simulink model "TCS5"  (R2018b)
settings: Solver=VariableStepAuto  StartTime=0.0  StopTime=10  RelTol=1e-3
model workspace (MAT data in the model file):
  Ki = Simulink.Parameter
  Ki.Value = 50000
  Ki.Description = 'PID积分系数'
  Ki.DataType = 'auto'
  Ki.Dimensions = [1 1]
  Kp = Simulink.Parameter
  Kp.Value = 40000
  Kp.Description = 'PID比例系数'
  Kp.DataType = 'auto'
  Kp.Dimensions = [1 1]
  T_max = Simulink.Parameter
  T_max.Value = 10000
  T_max.Description = '电机最大转矩'
  T_max.DataType = 'auto'
  T_max.Dimensions = [1 1]
  Vobj = Simulink.Parameter
  Vobj.Value = 40
  Vobj.DataType = 'auto'
  Vobj.Dimensions = [1 1]
  r = Simulink.Parameter
  r.Value = 0.538
  r.Description = '车轮滚动半径'
  r.DataType = 'auto'
  r.Dimensions = [1 1]
  s_obj = Simulink.Parameter
  s_obj.Value = 0.13
  s_obj.DataType = 'auto'
  s_obj.Dimensions = [1 1]
undefined symbols (not defined in the file): DiscIntNeverNeededParam
libraries: simulink x8, Solver_SF x1
(part 1 of 2)
settings Model: OrderedModelArguments=off  Creator=14615  LastModifiedBy=14615
settings DataIOCC: ReturnWorkspaceOutputs=on
settings DebuggingCC: SFMachineParentedDataDiag=error

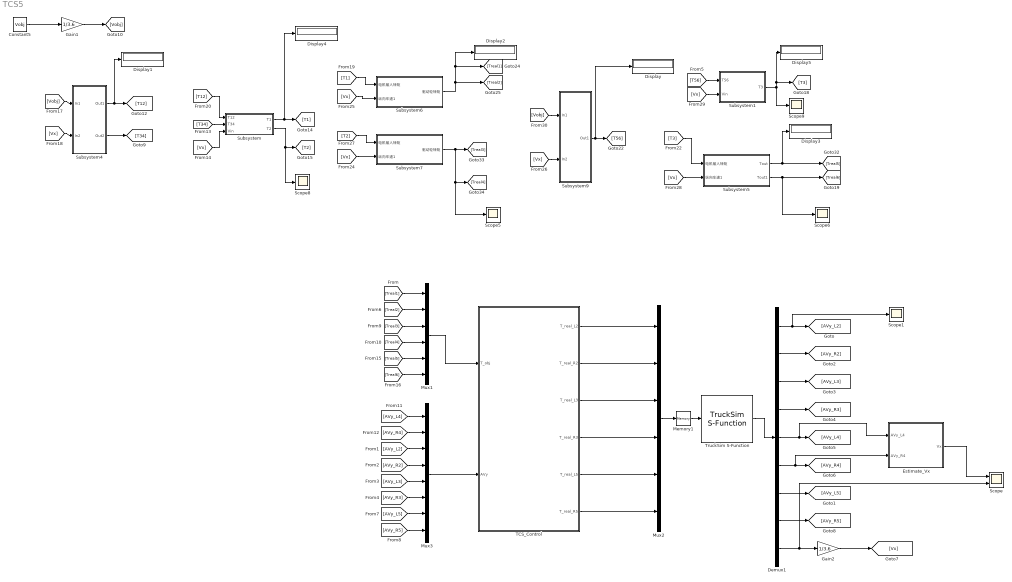
== system TCS5 ==
  Constant5 : Constant  Value=Vobj
  Demux1 : Demux  Outputs=9
  Display{,1..5} (6 alike) : Display
  Estimate_Vx : Subsystem
  Gain1 : Gain  Gain=1/3.6
  Gain2 : Gain  Gain=1/3.6
  Memory1 : Memory
  Mux1 : Mux  Inputs=6
  Mux2 : Mux  Inputs=6
  Mux3 : Mux  Inputs=8
  Scope : Scope  NumInputPorts=2
  Scope{1,5..6,8..9} (5 alike) : Scope
  Subsystem : Subsystem
  Subsystem1 : Subsystem
  Subsystem4 : Subsystem
  Subsystem5 : Subsystem
  Subsystem6 : Subsystem
  Subsystem7 : Subsystem
  Subsystem9 : Subsystem
  TCS_Control : Subsystem
  TruckSim S-Function : Solver_SF/TruckSim S-Function  Priority=1  SIMFILE=simfile.sim
  wires:
  Mux1/1 -> TCS_Control/1(T_obj)
  Mux2/1 -> Memory1/1
  TruckSim S-Function/1 -> Demux1/1
  Memory1/1 -> TruckSim S-Function/1
  Mux3/1 -> TCS_Control/2(AVy)
  [Treal1] -> Mux1/1
  [Treal6] -> Mux1/6
  [Treal4] -> Mux1/4
  [Treal3] -> Mux1/3
  [Treal2] -> Mux1/2
  [Treal5] -> Mux1/5
  [AVy_L4] -> Mux3/1
  [AVy_R4] -> Mux3/2
  [AVy_L2] -> Mux3/3
  [AVy_R2] -> Mux3/4
  [AVy_L3] -> Mux3/5
  [AVy_R3] -> Mux3/6
  [AVy_L5] -> Mux3/7
  [AVy_R5] -> Mux3/8
  TCS_Control/2(T_real_R2) -> Mux2/2
  TCS_Control/3(T_real_L3) -> Mux2/3
  TCS_Control/1(T_real_L2) -> Mux2/1
  TCS_Control/4(T_real_R3) -> Mux2/4
  Demux1/8 -> [AVy_R5]
  Demux1/6 -> Estimate_Vx/2(AVy_R4), [AVy_R4]
  Demux1/9 -> Scope/2, Gain2/1
  Estimate_Vx/1(Vx) -> Scope/1
  TCS_Control/5(T_real_L5) -> Mux2/5
  TCS_Control/6(T_real_R5) -> Mux2/6
  Subsystem/1(T1) -> Display4/1, [T1]
  [T1] -> Subsystem6/1(电机输入转矩)
  [Vobj] -> Subsystem9/1(In1)
  [T12] -> Subsystem/1(T12)
  Subsystem6/1(驱动轮转矩) -> [Treal2], [Treal1], Display2/1
  [T2] -> Subsystem7/1(电机输入转矩)
  [T3] -> Subsystem5/1(电机输入转矩)
  [Vobj] -> Subsystem4/1(In1)
  [T34] -> Subsystem/2(T34)
  Subsystem5/1(Tout) -> Display3/1, [Treal5]
  Subsystem4/1(Out1) -> Display1/1, [T12]
  Subsystem9/1(Out1) -> Display/1, [T56]
  [Vx] -> Subsystem4/2(In2)
  [T56] -> Subsystem1/1(T56)
  Subsystem/2(T2) -> Scope8/1, [T2]
  Subsystem4/2(Out2) -> [T34]
  Subsystem5/2(Tout1) -> [Treal6], Scope6/1
  Subsystem7/1(驱动轮转矩) -> [Treal4], Scope5/1, [Treal3]
  [Vx] -> Subsystem7/2(纵向车速1)
  [Vx] -> Subsystem1/2(Vin)
  [Vx] -> Subsystem9/2(In2)
  [Vx] -> Subsystem/3(Vin)
  Constant5/1 -> Gain1/1
  Subsystem1/1(T3) -> Display5/1, [T3], Scope9/1
  [Vx] -> Subsystem6/2(纵向车速1)
  [Vx] -> Subsystem5/2(纵向车速1)
  Gain1/1 -> [Vobj]
  Gain2/1 -> [Vx]
  Demux1/1 -> Scope1/1, [AVy_L2]
  Demux1/2 -> [AVy_R2]
  Demux1/3 -> [AVy_L3]
  Demux1/4 -> [AVy_R3]
  Demux1/5 -> Estimate_Vx/1(AVy_L4), [AVy_L4]
  Demux1/7 -> [AVy_L5]

== system TCS5/Estimate_Vx ==
  AVy_L4 : Inport
  AVy_R4 : Inport  Port=2
  Add : Sum
  Gain : Gain  Gain=pi/30
  Gain1 : Gain  Gain=3.6
  Gain2 : Gain  Gain=pi/30
  Gain3 : Gain  Gain=3.6
  Gain4 : Gain  Gain=0.5
  Product : Product
  Product1 : Product
  轮胎滚动半径 : Constant  Value=r
  轮胎滚动半径1 : Constant  Value=r
  Vx : Outport
  wires:
  Gain/1 -> Product/1
  Product1/1 -> Gain3/1
  Gain3/1 -> Add/2
  轮胎滚动半径/1 -> Product/2
  轮胎滚动半径1/1 -> Product1/2
  Add/1 -> Gain4/1
  Gain4/1 -> Vx/1
  Product/1 -> Gain1/1
  Gain1/1 -> Add/1
  Gain2/1 -> Product1/1
  AVy_R4/1 -> Gain2/1
  AVy_L4/1 -> Gain/1

== system TCS5/Subsystem ==
  T12 : Inport
  T34 : Inport  Port=2
  Vin : Inport  Port=3
  Gain : Gain  Gain=3.6
  Product : Product  SaturateOnIntegerOverflow=on  InputSameDT=on  OutDataTypeStr=Inherit: Same as first input
  Product1 : Product  SaturateOnIntegerOverflow=on  InputSameDT=on  OutDataTypeStr=Inherit: Same as first input
  Saturation : Saturate  UpperLimit=2000  LowerLimit=-2000
  Saturation1 : Saturate  UpperLimit=2000  LowerLimit=-2000
  Table : Lookup_n-D  NumberOfTableDimensions=1  BreakpointsForDimension1=[1 2 3 4]  Table=[0.1261,0.2833,0.5747,1.00]  OutDataTypeStr=double  SaturateOnIntegerOverflow=on  InputSameDT=on  LockScale=on
  换挡逻辑 : Subsystem
  T1 : Outport  VectorParamsAs1DForOutWhenUnconnected=on
  T2 : Outport  Port=2  VectorParamsAs1DForOutWhenUnconnected=on
  wires:
  Vin/1 -> Gain/1
  换挡逻辑/1(gear) -> Table/1
  T12/1 -> Product/1
  Table/1 -> Product/2, Product1/1
  T34/1 -> Product1/2
  Gain/1 -> 换挡逻辑/1(v)
  Product1/1 -> Saturation/1
  Saturation/1 -> T2/1
  Product/1 -> Saturation1/1
  Saturation1/1 -> T1/1

== system TCS5/Subsystem1 ==
  T56 : Inport
  Vin : Inport  Port=2
  Gain : Gain  Gain=3.6
  Gain2 : Gain
  Product2 : Product  SaturateOnIntegerOverflow=on  InputSameDT=on  OutDataTypeStr=Inherit: Same as first input
  Saturation1 : Saturate  UpperLimit=2000  LowerLimit=-2000
  Table : Lookup_n-D  NumberOfTableDimensions=1  BreakpointsForDimension1=[1 2 3 4]  Table=[0.1261,0.2833,0.5747,1.00]  OutDataTypeStr=double  SaturateOnIntegerOverflow=on  InputSameDT=on  LockScale=on
  换挡逻辑 : Subsystem
  T3 : Outport  VectorParamsAs1DForOutWhenUnconnected=on
  wires:
  换挡逻辑/1(gear) -> Table/1
  Vin/1 -> Gain/1
  Table/1 -> Product2/1
  T56/1 -> Product2/2
  Gain/1 -> 换挡逻辑/1(v)
  Product2/1 -> Saturation1/1
  Saturation1/1 -> Gain2/1
  Gain2/1 -> T3/1

== system TCS5/Subsystem4 ==
  In1 : Inport
  In2 : Inport  Port=2
  0.1 : simulink/Continuous/PID Controller  Controller=PID  Form=Parallel  TimeDomain=Discrete-time  SampleTime=-1  IntegratorMethod=Forward Euler  FilterMethod=Forward Euler  ControllerParametersSource=internal  P=10000  I=0  D=0  UseFilter=on  N=100  TunerSelectOption=Transfer Function Based (PID Tuner App)  InitialConditionSource=internal  InitialConditionForIntegrator=0  InitialConditionForFilter=0  DifferentiatorICPrevScaledInput=0  ExternalReset=none  TrackingMode=off  Kt=1  LimitOutput=off  UpperSaturationLimit=inf  LowerSaturationLimit=-inf  LinearizeAsGain=on  AntiWindupMode=none  Kb=1  POutMin=[]  POutMax=[]  IOutMin=[]  IOutMax=[]  DOutMin=[]  DOutMax=[]  NOutMin=[]  NOutMax=[]  SumOutMin=[]  SumOutMax=[]  SaturationOutMin=[]  SaturationOutMax=[]  PParamMin=[]  PParamMax=[]  IParamMin=[]  IParamMax=[]  DParamMin=[]  DParamMax=[]  NParamMin=[]  NParamMax=[]  KbParamMin=[]  KbParamMax=[]  KtParamMin=[]  KtParamMax=[]  KbOutMin=[]  KbOutMax=[]  KtOutMin=[]  KtOutMax=[]  IntegratorOutMin=[]  IntegratorOutMax=[]  FilterOutMin=[]  FilterOutMax=[]  SumI1OutMin=[]  SumI1OutMax=[]  SumI2OutMin=[]  SumI2OutMax=[]  SumI3OutMin=[]  SumI3OutMax=[]  SumI4OutMin=[]  SumI4OutMax=[]  SumDOutMin=[]  SumDOutMax=[]  DifferentiatorOutMin=[]  DifferentiatorOutMax=[]  FilterDiffOutCoefMin=[]  FilterDiffOutCoefMax=[]  ReciprocalOutMin=[]  ReciprocalOutMax=[]  SumDenOutMin=[]  SumDenOutMax=[]  SumNumOutMin=[]  SumNumOutMax=[]  DivideOutMin=[]  DivideOutMax=[]  IntegratorContinuousStateAttributes=''  IntegratorStateMustResolveToSignalObject=off  IntegratorRTWStateStorageClass=Auto  FilterContinuousStateAttributes=''  FilterStateMustResolveToSignalObject=off  FilterRTWStateStorageClass=Auto  ParallelPVariant=InternalParameters  IdealPVariant=Disabled  IVariant=InternalParameters  DVariant=InternalParameters  IntegratorVariant=Discrete  SatVariant=Disabled  AWVariant=Passthrough  PCopyVariant=Disabled  TRVariant=Disabled  FdbkBlocksVariant=Forward  IdealPFdbkVariant=Disabled  SatFdbkVariant=Disabled  DerivativeFilterVariant=ForwardEulerFilter  NVariant=InternalParameters  NCopyVariant=Disabled  FilterICVariant=InternalICsFilter  IntegratorICVariant=InternalICs  ExternalResetVariant=Disabled  TRSumVariant=Passthrough  SumFdbkVariant=Disabled  SumVariant=Sum_PID
  Fcn : Fcn  Expr=u(1)*u(2)/4
  Mux : Mux  Inputs=2
  R : Constant  Value=0.538
  Sum : Sum  Inputs=|+-
  Out1 : Outport  VectorParamsAs1DForOutWhenUnconnected=on
  Out2 : Outport  Port=2  VectorParamsAs1DForOutWhenUnconnected=on
  wires:
  0.1/1 -> Mux/1
  Fcn/1 -> Out2/1, Out1/1
  Sum/1 -> 0.1/1
  In1/1 -> Sum/1
  In2/1 -> Sum/2
  R/1 -> Mux/2
  Mux/1 -> Fcn/1

== system TCS5/Subsystem5 ==
  电机输入转矩 : Inport
  纵向车速1 : Inport  Port=2
  Gain : Gain  Gain=3.6
  PMSM : Subsystem  mask{pp=4, Rs=0.05, Jm=0.008, ld=0.0001, lq=0.0001, flux=0.17, f=1.349e-5}
      mask prompts: pp "极对数"; Rs "定子电阻"; Jm "转动惯量"; ld "d轴电感"; lq "q轴电感"; flux "永磁体磁链"; f "粘性阻尼"
  Product : Product
  SOC : Scope
  Subsystem : Subsystem
  充电电流 : Scope
  单位三相电 : Sin  Frequency=400*pi  Phase=[0 -2*pi/3 2*pi/3]  SampleTime=0
  变速器模型 : Subsystem
  差速器 : Gain  Gain=1/2
  换挡逻辑 : Subsystem
  电机输入\输出转矩 : Scope  NumInputPorts=2
  能量变化 : Scope
  驱动轮的转矩 : Scope
  Tout : Outport  VectorParamsAs1DForOutWhenUnconnected=on
  Tout1 : Outport  Port=2  VectorParamsAs1DForOutWhenUnconnected=on
  wires:
  差速器/1 -> Tout1/1, Tout/1, 驱动轮的转矩/1
  电机输入转矩/1 -> 电机输入\输出转矩/1, PMSM/1(Tm)
  换挡逻辑/1(gear) -> 变速器模型/2(Gear)
  变速器模型/1(Tout) -> 差速器/1
  Subsystem/1(能量变化) -> 能量变化/1
  PMSM/1(Te) -> 电机输入\输出转矩/2, 变速器模型/1(Tin)
  纵向车速1/1 -> Gain/1
  Product/1 -> PMSM/2(Uabc)
  单位三相电/1 -> Product/2
  Subsystem/3(输出电压V) -> Product/1
  PMSM/2(iq) -> 充电电流/1, Subsystem/1(充电电流A)
  Subsystem/2(SOC) -> SOC/1
  Gain/1 -> 换挡逻辑/1(v)

== system TCS5/Subsystem6 ==
  电机输入转矩 : Inport
  纵向车速1 : Inport  Port=2
  Gain : Gain  Gain=3.6
  PMSM : Subsystem  mask{pp=4, Rs=0.05, Jm=0.008, ld=0.0001, lq=0.0001, flux=0.17, f=1.349e-5}
      mask prompts: pp "极对数"; Rs "定子电阻"; Jm "转动惯量"; ld "d轴电感"; lq "q轴电感"; flux "永磁体磁链"; f "粘性阻尼"
  Product : Product
  SOC : Scope
  Subsystem : Subsystem
  充电电流 : Scope
  单位三相电 : Sin  Frequency=400*pi  Phase=[0 -2*pi/3 2*pi/3]  SampleTime=0
  变速器模型 : Subsystem
  差速器 : Gain  Gain=1/2
  换挡逻辑 : Subsystem
  能量变化 : Scope
  驱动轮的转矩 : Scope
  驱动轮转矩 : Outport  VectorParamsAs1DForOutWhenUnconnected=on
  wires:
  Product/1 -> PMSM/2(Uabc)
  电机输入转矩/1 -> PMSM/1(Tm)
  变速器模型/1(Tout) -> 差速器/1
  Subsystem/2(SOC) -> SOC/1
  纵向车速1/1 -> Gain/1
  换挡逻辑/1(gear) -> 变速器模型/2(Gear)
  PMSM/1(Te) -> 变速器模型/1(Tin)
  Subsystem/3(输出电压V) -> Product/1
  单位三相电/1 -> Product/2
  PMSM/2(iq) -> 充电电流/1, Subsystem/1(充电电流A)
  差速器/1 -> 驱动轮的转矩/1, 驱动轮转矩/1
  Subsystem/1(能量变化) -> 能量变化/1
  Gain/1 -> 换挡逻辑/1(v)

== system TCS5/Subsystem7 ==
  电机输入转矩 : Inport
  纵向车速1 : Inport  Port=2
  Gain : Gain  Gain=3.6
  PMSM : Subsystem  mask{pp=4, Rs=0.05, Jm=0.008, ld=0.0001, lq=0.0001, flux=0.17, f=1.349e-5}
      mask prompts: pp "极对数"; Rs "定子电阻"; Jm "转动惯量"; ld "d轴电感"; lq "q轴电感"; flux "永磁体磁链"; f "粘性阻尼"
  Product : Product
  SOC : Scope
  Subsystem : Subsystem
  充电电流 : Scope
  单位三相电 : Sin  Frequency=400*pi  Phase=[0 -2*pi/3 2*pi/3]  SampleTime=0
  变速器模型 : Subsystem
  差速器 : Gain  Gain=1/2
  换挡逻辑 : Subsystem
  电机输入\输出转矩 : Scope  NumInputPorts=2
  能量变化 : Scope
  驱动轮的转矩 : Scope
  驱动轮转矩 : Outport  VectorParamsAs1DForOutWhenUnconnected=on
  wires:
  电机输入转矩/1 -> 电机输入\输出转矩/1, PMSM/1(Tm)
  换挡逻辑/1(gear) -> 变速器模型/2(Gear)
  变速器模型/1(Tout) -> 差速器/1
  Subsystem/1(能量变化) -> 能量变化/1
  PMSM/1(Te) -> 电机输入\输出转矩/2, 变速器模型/1(Tin)
  纵向车速1/1 -> Gain/1
  Product/1 -> PMSM/2(Uabc)
  单位三相电/1 -> Product/2
  Subsystem/3(输出电压V) -> Product/1
  PMSM/2(iq) -> 充电电流/1, Subsystem/1(充电电流A)
  Subsystem/2(SOC) -> SOC/1
  差速器/1 -> 驱动轮的转矩/1, 驱动轮转矩/1
  Gain/1 -> 换挡逻辑/1(v)

== system TCS5/Subsystem9 ==
  In1 : Inport
  In2 : Inport  Port=2
  0.1 : simulink/Continuous/PID Controller  Controller=PID  Form=Parallel  TimeDomain=Discrete-time  SampleTime=-1  IntegratorMethod=Forward Euler  FilterMethod=Forward Euler  ControllerParametersSource=internal  P=10000  I=0  D=0  UseFilter=on  N=100  TunerSelectOption=Transfer Function Based (PID Tuner App)  InitialConditionSource=internal  InitialConditionForIntegrator=0  InitialConditionForFilter=0  DifferentiatorICPrevScaledInput=0  ExternalReset=none  TrackingMode=off  Kt=1  LimitOutput=off  UpperSaturationLimit=inf  LowerSaturationLimit=-inf  LinearizeAsGain=on  AntiWindupMode=none  Kb=1  POutMin=[]  POutMax=[]  IOutMin=[]  IOutMax=[]  DOutMin=[]  DOutMax=[]  NOutMin=[]  NOutMax=[]  SumOutMin=[]  SumOutMax=[]  SaturationOutMin=[]  SaturationOutMax=[]  PParamMin=[]  PParamMax=[]  IParamMin=[]  IParamMax=[]  DParamMin=[]  DParamMax=[]  NParamMin=[]  NParamMax=[]  KbParamMin=[]  KbParamMax=[]  KtParamMin=[]  KtParamMax=[]  KbOutMin=[]  KbOutMax=[]  KtOutMin=[]  KtOutMax=[]  IntegratorOutMin=[]  IntegratorOutMax=[]  FilterOutMin=[]  FilterOutMax=[]  SumI1OutMin=[]  SumI1OutMax=[]  SumI2OutMin=[]  SumI2OutMax=[]  SumI3OutMin=[]  SumI3OutMax=[]  SumI4OutMin=[]  SumI4OutMax=[]  SumDOutMin=[]  SumDOutMax=[]  DifferentiatorOutMin=[]  DifferentiatorOutMax=[]  FilterDiffOutCoefMin=[]  FilterDiffOutCoefMax=[]  ReciprocalOutMin=[]  ReciprocalOutMax=[]  SumDenOutMin=[]  SumDenOutMax=[]  SumNumOutMin=[]  SumNumOutMax=[]  DivideOutMin=[]  DivideOutMax=[]  IntegratorContinuousStateAttributes=''  IntegratorStateMustResolveToSignalObject=off  IntegratorRTWStateStorageClass=Auto  FilterContinuousStateAttributes=''  FilterStateMustResolveToSignalObject=off  FilterRTWStateStorageClass=Auto  ParallelPVariant=InternalParameters  IdealPVariant=Disabled  IVariant=InternalParameters  DVariant=InternalParameters  IntegratorVariant=Discrete  SatVariant=Disabled  AWVariant=Passthrough  PCopyVariant=Disabled  TRVariant=Disabled  FdbkBlocksVariant=Forward  IdealPFdbkVariant=Disabled  SatFdbkVariant=Disabled  DerivativeFilterVariant=ForwardEulerFilter  NVariant=InternalParameters  NCopyVariant=Disabled  FilterICVariant=InternalICsFilter  IntegratorICVariant=InternalICs  ExternalResetVariant=Disabled  TRSumVariant=Passthrough  SumFdbkVariant=Disabled  SumVariant=Sum_PID
  Fcn : Fcn  Expr=u(1)*u(2)/4
  Mux : Mux  Inputs=2
  R : Constant  Value=0.538
  Sum : Sum  Inputs=|+-
  Out1 : Outport  VectorParamsAs1DForOutWhenUnconnected=on
  wires:
  0.1/1 -> Mux/1
  Sum/1 -> 0.1/1
  In1/1 -> Sum/1
  Fcn/1 -> Out1/1
  In2/1 -> Sum/2
  R/1 -> Mux/2
  Mux/1 -> Fcn/1

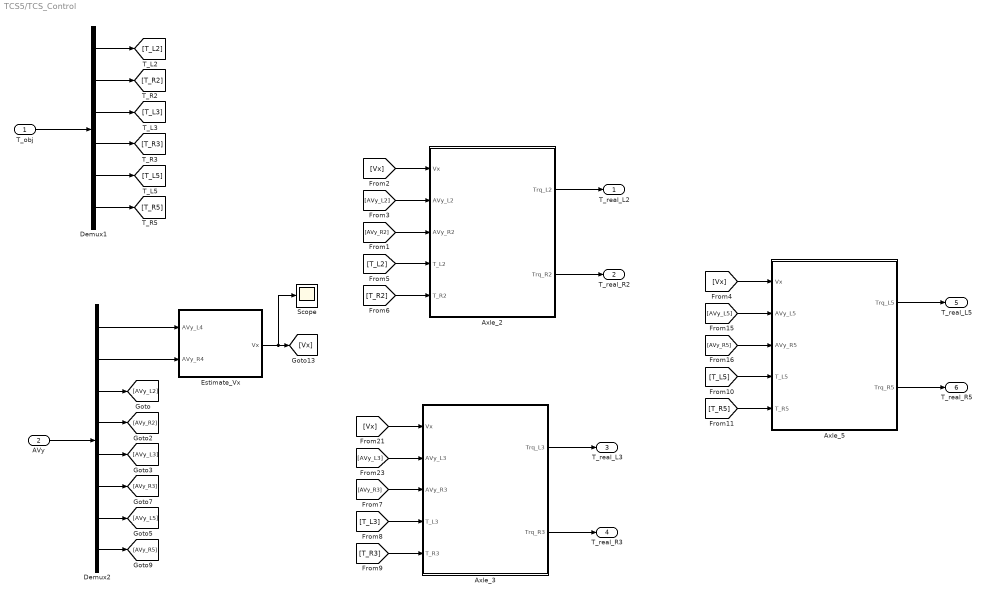
== system TCS5/TCS_Control ==
  T_obj : Inport
  AVy : Inport  Port=2
  Axle_2 : Subsystem
  Axle_3 : Subsystem
  Axle_5 : Subsystem
  Demux1 : Demux  Outputs=6
  Demux2 : Demux  Outputs=8
  Estimate_Vx : Subsystem
  Scope : Scope
  T_real_L2 : Outport
  T_real_R2 : Outport  Port=2
  T_real_L3 : Outport  Port=3
  T_real_R3 : Outport  Port=4
  T_real_L5 : Outport  Port=5
  T_real_R5 : Outport  Port=6
  wires:
  T_obj/1 -> Demux1/1
  Demux1/5 -> [T_L5]
  Demux1/6 -> [T_R5]
  AVy/1 -> Demux2/1
  [AVy_L2] -> Axle_2/2(AVy_L2)
  [AVy_R2] -> Axle_2/3(AVy_R2)
  [Vx] -> Axle_2/1(Vx)
  [T_L2] -> Axle_2/4(T_L2)
  [T_R2] -> Axle_2/5(T_R2)
  Axle_2/1(Trq_L2) -> T_real_L2/1
  Axle_2/2(Trq_R2) -> T_real_R2/1
  [T_L3] -> Axle_3/4(T_L3)
  Axle_3/2(Trq_R3) -> T_real_R3/1
  [AVy_L3] -> Axle_3/2(AVy_L3)
  [Vx] -> Axle_3/1(Vx)
  Axle_3/1(Trq_L3) -> T_real_L3/1
  [AVy_R3] -> Axle_3/3(AVy_R3)
  [T_R3] -> Axle_3/5(T_R3)
  [AVy_L5] -> Axle_5/2(AVy_L5)
  [T_R5] -> Axle_5/5(T_R5)
  [Vx] -> Axle_5/1(Vx)
  [AVy_R5] -> Axle_5/3(AVy_R5)
  [T_L5] -> Axle_5/4(T_L5)
  Demux1/1 -> [T_L2]
  Demux1/2 -> [T_R2]
  Demux1/3 -> [T_L3]
  Demux1/4 -> [T_R3]
  Demux2/3 -> [AVy_L2]
  Demux2/4 -> [AVy_R2]
  Demux2/5 -> [AVy_L3]
  Demux2/6 -> [AVy_R3]
  Demux2/7 -> [AVy_L5]
  Demux2/8 -> [AVy_R5]
  Estimate_Vx/1(Vx) -> Scope/1, [Vx]
  Demux2/1 -> Estimate_Vx/1(AVy_L4)
  Demux2/2 -> Estimate_Vx/2(AVy_R4)
  Axle_5/1(Trq_L5) -> T_real_L5/1
  Axle_5/2(Trq_R5) -> T_real_R5/1

== system TCS5/Subsystem/换挡逻辑 ==
  v : Inport
  Constant3 : Constant  Value=0
  Constant4 : Constant  Value=0
  Constant5 : Constant  Value=0
  Constant6 : Constant
  Rocker Switch : RockerSwitchBlock  WebBlockId=2223
      settings: Values={{'Off', 'On'}, [0 1]}
  Rocker Switch1 : RockerSwitchBlock  WebBlockId=2224
      settings: Values={{'Off', 'On'}, [0 1]}
  Rocker Switch2 : RockerSwitchBlock  WebBlockId=2225
      settings: Values={{'Off', 'On'}, [0 1]}
  Rocker Switch3 : RockerSwitchBlock  WebBlockId=2226
      settings: Values={{'Off', 'On'}, [0 1]}
  "换档策略 " : Stateflow chart  TreatAsAtomicUnit=on
  gear : Outport  VectorParamsAs1DForOutWhenUnconnected=on
  wires:
  Constant3/1 -> "换档策略 "/2(PP)
  Constant6/1 -> "换档策略 "/5(DD)
  "换档策略 "/1(gear) -> gear/1
  Constant4/1 -> "换档策略 "/3(RR)
  Constant5/1 -> "换档策略 "/4(NN)
  v/1 -> "换档策略 "/1(v)

== system TCS5/Subsystem1/换挡逻辑 ==
  v : Inport
  Constant3 : Constant  Value=0
  Constant4 : Constant  Value=0
  Constant5 : Constant  Value=0
  Constant6 : Constant
  Rocker Switch : RockerSwitchBlock  WebBlockId=2245
      settings: Values={{'Off', 'On'}, [0 1]}
  Rocker Switch1 : RockerSwitchBlock  WebBlockId=2246
      settings: Values={{'Off', 'On'}, [0 1]}
  Rocker Switch2 : RockerSwitchBlock  WebBlockId=2247
      settings: Values={{'Off', 'On'}, [0 1]}
  Rocker Switch3 : RockerSwitchBlock  WebBlockId=2248
      settings: Values={{'Off', 'On'}, [0 1]}
  "换档策略 " : Stateflow chart  TreatAsAtomicUnit=on
  gear : Outport  VectorParamsAs1DForOutWhenUnconnected=on
  wires:
  Constant6/1 -> "换档策略 "/5(DD)
  Constant4/1 -> "换档策略 "/3(RR)
  "换档策略 "/1(gear) -> gear/1
  v/1 -> "换档策略 "/1(v)
  Constant5/1 -> "换档策略 "/4(NN)
  Constant3/1 -> "换档策略 "/2(PP)

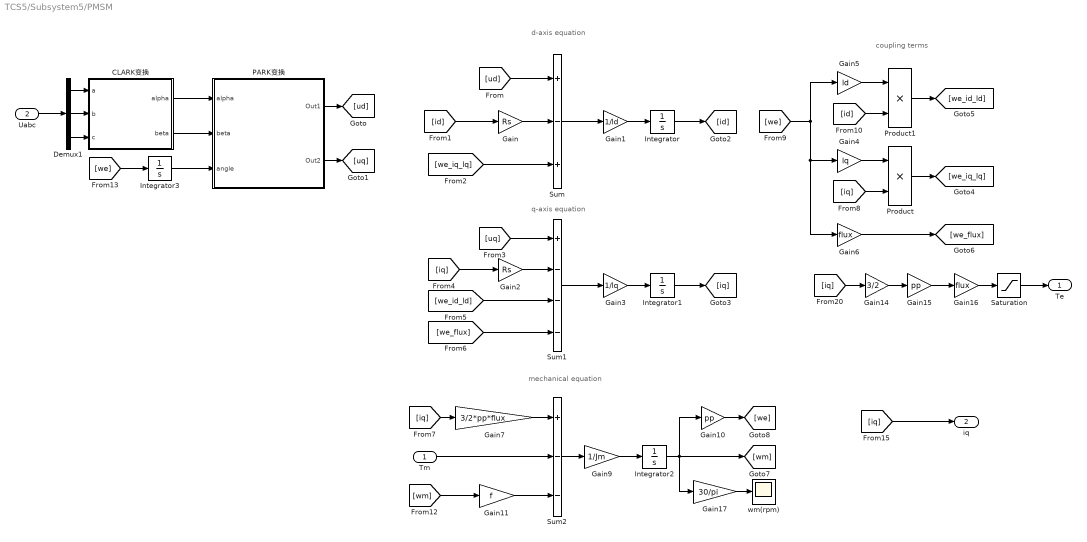
== system TCS5/Subsystem5/PMSM ==
  note: d-axis equation
  note: coupling terms
  note: q-axis equation
  note: mechanical equation
  Tm : Inport
  Uabc : Inport  Port=2
  CLARK变换 : Subsystem
  Demux1 : Demux  Outputs=3
  Gain : Gain  Gain=Rs
  Gain1 : Gain  Gain=1/ld
  Gain10 : Gain  Gain=pp
  Gain11 : Gain  Gain=f
  Gain14 : Gain  Gain=3/2
  Gain15 : Gain  Gain=pp
  Gain16 : Gain  Gain=flux
  Gain17 : Gain  Gain=30/pi
  Gain2 : Gain  Gain=Rs
  Gain3 : Gain  Gain=1/lq
  Gain4 : Gain  Gain=lq
  Gain5 : Gain  Gain=ld
  Gain6 : Gain  Gain=flux
  Gain7 : Gain  Gain=3/2*pp*flux
  Gain9 : Gain  Gain=1/Jm
  Integrator{,1..3} (4 alike) : Integrator
  PARK变换 : Subsystem
  Product : Product
  Product1 : Product
  Saturation : Saturate  UpperLimit=2000  LowerLimit=-2000
  Sum : Sum  Inputs=+-+
  Sum1 : Sum  Inputs=+---
  Sum2 : Sum  Inputs=+--
  wm(rpm) : Scope
  Te : Outport
  iq : Outport  Port=2
  wires:
  [iq] -> Product/2
  Integrator2/1 -> Gain17/1, [wm], Gain10/1
  [we_iq_lq] -> Sum/3
  [iq] -> Gain7/1
  Product1/1 -> [we_id_ld]
  Sum/1 -> Gain1/1
  Gain1/1 -> Integrator/1
  Gain2/1 -> Sum1/2
  Gain5/1 -> Product1/1
  Gain/1 -> Sum/2
  Gain3/1 -> Integrator1/1
  Sum1/1 -> Gain3/1
  [id] -> Product1/2
  Tm/1 -> Sum2/2
  [iq] -> Gain2/1
  Gain6/1 -> [we_flux]
  Gain9/1 -> Integrator2/1
  Product/1 -> [we_iq_lq]
  Gain7/1 -> Sum2/1
  Integrator1/1 -> [iq]
  Sum2/1 -> Gain9/1
  Gain4/1 -> Product/1
  [ud] -> Sum/1
  Gain10/1 -> [we]
  [we_flux] -> Sum1/4
  [we_id_ld] -> Sum1/3
  [we] -> Gain4/1, Gain6/1, Gain5/1
  [id] -> Gain/1
  [uq] -> Sum1/1
  Gain11/1 -> Sum2/3
  [wm] -> Gain11/1
  [iq] -> Gain14/1
  Gain14/1 -> Gain15/1
  Gain15/1 -> Gain16/1
  Gain17/1 -> wm(rpm)/1
  Integrator/1 -> [id]
  [iq] -> iq/1
  Gain16/1 -> Saturation/1
  Saturation/1 -> Te/1
  Demux1/1 -> CLARK变换/1(a)
  Uabc/1 -> Demux1/1
  Demux1/3 -> CLARK变换/3(c)
  Demux1/2 -> CLARK变换/2(b)
  CLARK变换/1(alpha) -> PARK变换/1(alpha)
  CLARK变换/2(beta) -> PARK变换/2(beta)
  [we] -> Integrator3/1
  Integrator3/1 -> PARK变换/3(angle)
  PARK变换/1(Out1) -> [ud]
  PARK变换/2(Out2) -> [uq]

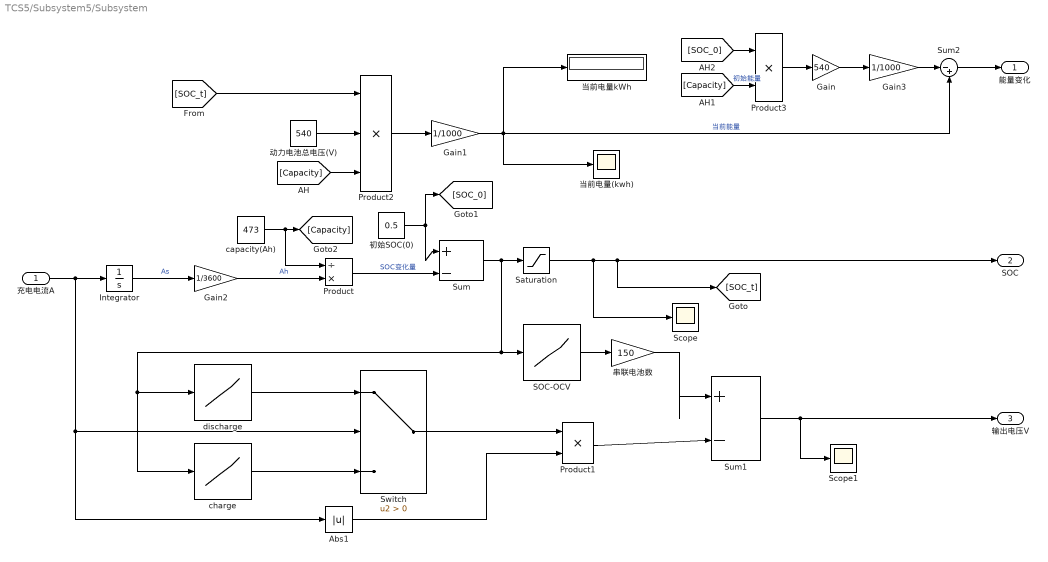
== system TCS5/Subsystem5/Subsystem ==
  充电电流A : Inport
  Abs1 : Abs
  Gain : Gain  Gain=540
  Gain1 : Gain  Gain=1/1000
  Gain2 : Gain  Gain=1/3600
  Gain3 : Gain  Gain=1/1000
  Integrator : Integrator
  Product : Product  Inputs=/*
  Product1 : Product
  Product2 : Product  Inputs=3
  Product3 : Product
  SOC-OCV : Lookup_n-D  NumberOfTableDimensions=1  BreakpointsForDimension1=[0,0.1,0.2,0.4,0.6,0.8,1]  Table=[3.31144,3.54994000000000013,3.63898,3.72908,3.8329600000000004,3.9771199999999998,4.131880000000001]  InternalRulePriority=Speed  RndMeth=Simplest  InputSameDT=on
  Saturation : Saturate  UpperLimit=1  LowerLimit=0
  Scope : Scope
  Scope1 : Scope
  Sum : Sum  Inputs=|+-
  Sum1 : Sum  Inputs=|+-
  Sum2 : Sum  Inputs=|-+
  Switch : Switch  Criteria=u2 > Threshold
  capacity(Ah) : Constant  Value=473
  charge : Lookup_n-D  NumberOfTableDimensions=1  BreakpointsForDimension1=[0,0.1,0.2,0.4,0.6,0.8,1]  Table=[0.02536,0.012695,0.0080907,0.006409000000000001,0.006565,0.0071812,0.0074386]  InternalRulePriority=Speed  RndMeth=Simplest  InputSameDT=on
  discharge : Lookup_n-D  NumberOfTableDimensions=1  BreakpointsForDimension1=[0,0.1,0.2,0.4,0.6,0.8,1]  Table=[0.02536,0.012695,0.0080907,0.006409000000000001,0.006565,0.0071812,0.0074386]  InternalRulePriority=Speed  RndMeth=Simplest  InputSameDT=on
  串联电池数 : Gain  Gain=150
  初始SOC(0) : Constant  Value=0.5
  动力电池总电压(V) : Constant  Value=540
  当前电量(kwh) : Scope
  当前电量kWh : Display
  能量变化 : Outport
  SOC : Outport  Port=2
  输出电压V : Outport  Port=3
  wires:
  Product2/1 -> Gain1/1
  初始SOC(0)/1 -> [SOC_0], Sum/1
  Saturation/1 -> Scope/1, SOC/1, [SOC_t]
  动力电池总电压(V)/1 -> Product2/2
  Product1/1 -> Sum1/2
  串联电池数/1 -> Sum1/1
  capacity(Ah)/1 -> [Capacity], Product/1
  Sum1/1 -> 输出电压V/1, Scope1/1
  charge/1 -> Switch/3
  Gain1/1 -> Sum2/2, 当前电量kWh/1, 当前电量(kwh)/1  "当前能量"
  SOC-OCV/1 -> 串联电池数/1
  充电电流A/1 -> Integrator/1, Abs1/1, Switch/2
  Sum/1 -> charge/1, discharge/1, SOC-OCV/1, Saturation/1
  Switch/1 -> Product1/1
  discharge/1 -> Switch/1
  [SOC_t] -> Product2/1
  Abs1/1 -> Product1/2
  [Capacity] -> Product2/3
  Product/1 -> Sum/2  "SOC变化量"
  Gain2/1 -> Product/2  "Ah"
  Integrator/1 -> Gain2/1  "As"
  Sum2/1 -> 能量变化/1
  Gain/1 -> Gain3/1
  Gain3/1 -> Sum2/1
  Product3/1 -> Gain/1
  [SOC_0] -> Product3/1
  [Capacity] -> Product3/2  "初始能量"

== system TCS5/Subsystem5/变速器模型 ==
  Tin : Inport  Unit=ft*lbf@torque
  Gear : Inport  Port=2  Unit=1
  Product : Product  SaturateOnIntegerOverflow=on  InputSameDT=on  OutDataTypeStr=Inherit: Same as first input
  Table : Lookup_n-D  NumberOfTableDimensions=1  BreakpointsForDimension1=[1 2 3 4]  Table=[7.93,3.53,1.74,1.00]  OutDataTypeStr=double  SaturateOnIntegerOverflow=on  InputSameDT=on  LockScale=on
  Tout : Outport  Unit=ft*lbf@torque
  wires:
  Table/1 -> Product/2
  Product/1 -> Tout/1
  Tin/1 -> Product/1
  Gear/1 -> Table/1

== system TCS5/Subsystem5/换挡逻辑 ==
  v : Inport
  Constant3 : Constant  Value=0
  Constant4 : Constant  Value=0
  Constant5 : Constant  Value=0
  Constant6 : Constant
  Rocker Switch : RockerSwitchBlock  WebBlockId=2406
      settings: Values={{'Off', 'On'}, [0 1]}
  Rocker Switch1 : RockerSwitchBlock  WebBlockId=2407
      settings: Values={{'Off', 'On'}, [0 1]}
  Rocker Switch2 : RockerSwitchBlock  WebBlockId=2408
      settings: Values={{'Off', 'On'}, [0 1]}
  Rocker Switch3 : RockerSwitchBlock  WebBlockId=2409
      settings: Values={{'Off', 'On'}, [0 1]}
  "换档策略 " : Stateflow chart  TreatAsAtomicUnit=on
  gear : Outport  VectorParamsAs1DForOutWhenUnconnected=on
  wires:
  Constant3/1 -> "换档策略 "/2(PP)
  Constant6/1 -> "换档策略 "/5(DD)
  "换档策略 "/1(gear) -> gear/1
  Constant4/1 -> "换档策略 "/3(RR)
  Constant5/1 -> "换档策略 "/4(NN)
  v/1 -> "换档策略 "/1(v)

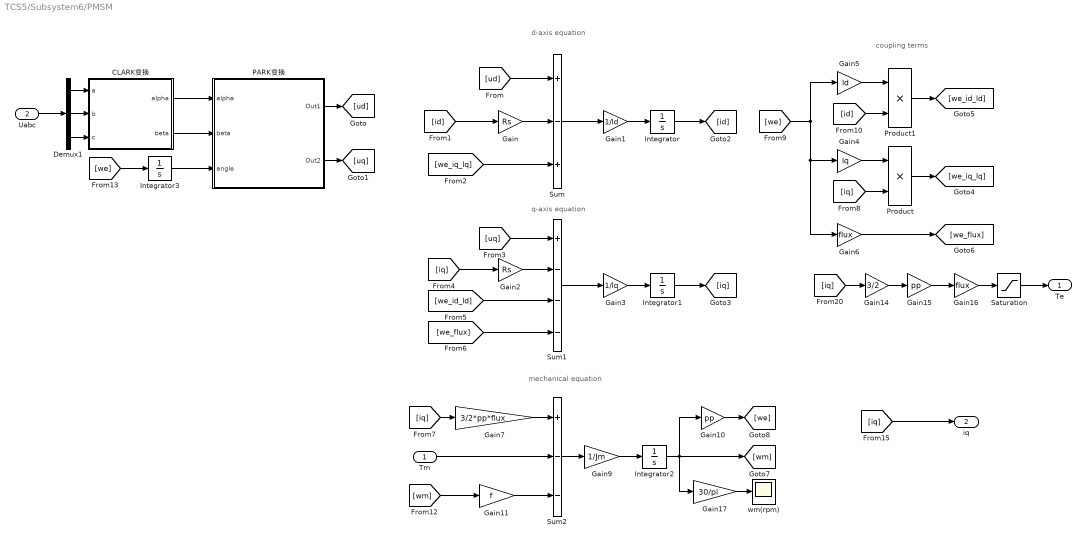
== system TCS5/Subsystem6/PMSM ==
  note: d-axis equation
  note: coupling terms
  note: q-axis equation
  note: mechanical equation
  Tm : Inport
  Uabc : Inport  Port=2
  CLARK变换 : Subsystem
  Demux1 : Demux  Outputs=3
  Gain : Gain  Gain=Rs
  Gain1 : Gain  Gain=1/ld
  Gain10 : Gain  Gain=pp
  Gain11 : Gain  Gain=f
  Gain14 : Gain  Gain=3/2
  Gain15 : Gain  Gain=pp
  Gain16 : Gain  Gain=flux
  Gain17 : Gain  Gain=30/pi
  Gain2 : Gain  Gain=Rs
  Gain3 : Gain  Gain=1/lq
  Gain4 : Gain  Gain=lq
  Gain5 : Gain  Gain=ld
  Gain6 : Gain  Gain=flux
  Gain7 : Gain  Gain=3/2*pp*flux
  Gain9 : Gain  Gain=1/Jm
  Integrator{,1..3} (4 alike) : Integrator
  PARK变换 : Subsystem
  Product : Product
  Product1 : Product
  Saturation : Saturate  UpperLimit=2000  LowerLimit=-2000
  Sum : Sum  Inputs=+-+
  Sum1 : Sum  Inputs=+---
  Sum2 : Sum  Inputs=+--
  wm(rpm) : Scope
  Te : Outport
  iq : Outport  Port=2
  wires:
  [iq] -> Product/2
  Integrator2/1 -> Gain17/1, [wm], Gain10/1
  [we_iq_lq] -> Sum/3
  [iq] -> Gain7/1
  Product1/1 -> [we_id_ld]
  Sum/1 -> Gain1/1
  Gain1/1 -> Integrator/1
  Gain2/1 -> Sum1/2
  Gain5/1 -> Product1/1
  Gain/1 -> Sum/2
  Gain3/1 -> Integrator1/1
  Sum1/1 -> Gain3/1
  [id] -> Product1/2
  Tm/1 -> Sum2/2
  [iq] -> Gain2/1
  Gain6/1 -> [we_flux]
  Gain9/1 -> Integrator2/1
  Product/1 -> [we_iq_lq]
  Gain7/1 -> Sum2/1
  Integrator1/1 -> [iq]
  Sum2/1 -> Gain9/1
  Gain4/1 -> Product/1
  [ud] -> Sum/1
  Gain10/1 -> [we]
  [we_flux] -> Sum1/4
  [we_id_ld] -> Sum1/3
  [we] -> Gain4/1, Gain6/1, Gain5/1
  [id] -> Gain/1
  [uq] -> Sum1/1
  Gain11/1 -> Sum2/3
  [wm] -> Gain11/1
  [iq] -> Gain14/1
  Gain14/1 -> Gain15/1
  Gain15/1 -> Gain16/1
  Gain17/1 -> wm(rpm)/1
  Integrator/1 -> [id]
  [iq] -> iq/1
  Gain16/1 -> Saturation/1
  Saturation/1 -> Te/1
  Demux1/1 -> CLARK变换/1(a)
  Uabc/1 -> Demux1/1
  Demux1/3 -> CLARK变换/3(c)
  Demux1/2 -> CLARK变换/2(b)
  CLARK变换/1(alpha) -> PARK变换/1(alpha)
  CLARK变换/2(beta) -> PARK变换/2(beta)
  [we] -> Integrator3/1
  Integrator3/1 -> PARK变换/3(angle)
  PARK变换/1(Out1) -> [ud]
  PARK变换/2(Out2) -> [uq]

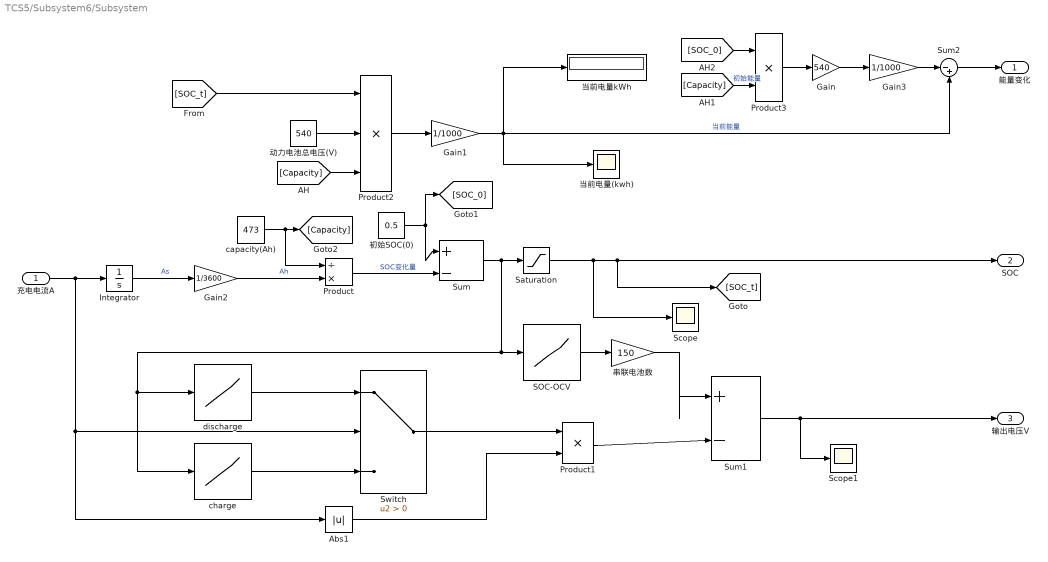
== system TCS5/Subsystem6/Subsystem ==
  充电电流A : Inport
  Abs1 : Abs
  Gain : Gain  Gain=540
  Gain1 : Gain  Gain=1/1000
  Gain2 : Gain  Gain=1/3600
  Gain3 : Gain  Gain=1/1000
  Integrator : Integrator
  Product : Product  Inputs=/*
  Product1 : Product
  Product2 : Product  Inputs=3
  Product3 : Product
  SOC-OCV : Lookup_n-D  NumberOfTableDimensions=1  BreakpointsForDimension1=[0,0.1,0.2,0.4,0.6,0.8,1]  Table=[3.31144,3.54994000000000013,3.63898,3.72908,3.8329600000000004,3.9771199999999998,4.131880000000001]  InternalRulePriority=Speed  RndMeth=Simplest  InputSameDT=on
  Saturation : Saturate  UpperLimit=1  LowerLimit=0
  Scope : Scope
  Scope1 : Scope
  Sum : Sum  Inputs=|+-
  Sum1 : Sum  Inputs=|+-
  Sum2 : Sum  Inputs=|-+
  Switch : Switch  Criteria=u2 > Threshold
  capacity(Ah) : Constant  Value=473
  charge : Lookup_n-D  NumberOfTableDimensions=1  BreakpointsForDimension1=[0,0.1,0.2,0.4,0.6,0.8,1]  Table=[0.02536,0.012695,0.0080907,0.006409000000000001,0.006565,0.0071812,0.0074386]  InternalRulePriority=Speed  RndMeth=Simplest  InputSameDT=on
  discharge : Lookup_n-D  NumberOfTableDimensions=1  BreakpointsForDimension1=[0,0.1,0.2,0.4,0.6,0.8,1]  Table=[0.02536,0.012695,0.0080907,0.006409000000000001,0.006565,0.0071812,0.0074386]  InternalRulePriority=Speed  RndMeth=Simplest  InputSameDT=on
  串联电池数 : Gain  Gain=150
  初始SOC(0) : Constant  Value=0.5
  动力电池总电压(V) : Constant  Value=540
  当前电量(kwh) : Scope
  当前电量kWh : Display
  能量变化 : Outport
  SOC : Outport  Port=2
  输出电压V : Outport  Port=3
  wires:
  Product2/1 -> Gain1/1
  初始SOC(0)/1 -> [SOC_0], Sum/1
  Saturation/1 -> Scope/1, SOC/1, [SOC_t]
  动力电池总电压(V)/1 -> Product2/2
  Product1/1 -> Sum1/2
  串联电池数/1 -> Sum1/1
  capacity(Ah)/1 -> [Capacity], Product/1
  Sum1/1 -> 输出电压V/1, Scope1/1
  charge/1 -> Switch/3
  Gain1/1 -> Sum2/2, 当前电量kWh/1, 当前电量(kwh)/1  "当前能量"
  SOC-OCV/1 -> 串联电池数/1
  充电电流A/1 -> Integrator/1, Abs1/1, Switch/2
  Sum/1 -> charge/1, discharge/1, SOC-OCV/1, Saturation/1
  Switch/1 -> Product1/1
  discharge/1 -> Switch/1
  [SOC_t] -> Product2/1
  Abs1/1 -> Product1/2
  [Capacity] -> Product2/3
  Product/1 -> Sum/2  "SOC变化量"
  Gain2/1 -> Product/2  "Ah"
  Integrator/1 -> Gain2/1  "As"
  Sum2/1 -> 能量变化/1
  Gain/1 -> Gain3/1
  Gain3/1 -> Sum2/1
  Product3/1 -> Gain/1
  [SOC_0] -> Product3/1
  [Capacity] -> Product3/2  "初始能量"

== system TCS5/Subsystem6/变速器模型 ==
  Tin : Inport  Unit=ft*lbf@torque
  Gear : Inport  Port=2  Unit=1
  Product : Product  SaturateOnIntegerOverflow=on  InputSameDT=on  OutDataTypeStr=Inherit: Same as first input
  Table : Lookup_n-D  NumberOfTableDimensions=1  BreakpointsForDimension1=[1 2 3 4]  Table=[7.93,3.53,1.74,1.00]  OutDataTypeStr=double  SaturateOnIntegerOverflow=on  InputSameDT=on  LockScale=on
  Tout : Outport  Unit=ft*lbf@torque
  wires:
  Table/1 -> Product/2
  Product/1 -> Tout/1
  Tin/1 -> Product/1
  Gear/1 -> Table/1

== system TCS5/Subsystem6/换挡逻辑 ==
  v : Inport
  Constant3 : Constant  Value=0
  Constant4 : Constant  Value=0
  Constant5 : Constant  Value=0
  Constant6 : Constant
  Rocker Switch : RockerSwitchBlock  WebBlockId=2554
      settings: Values={{'Off', 'On'}, [0 1]}
  Rocker Switch1 : RockerSwitchBlock  WebBlockId=2555
      settings: Values={{'Off', 'On'}, [0 1]}
  Rocker Switch2 : RockerSwitchBlock  WebBlockId=2556
      settings: Values={{'Off', 'On'}, [0 1]}
  Rocker Switch3 : RockerSwitchBlock  WebBlockId=2557
      settings: Values={{'Off', 'On'}, [0 1]}
  "换档策略 " : Stateflow chart  TreatAsAtomicUnit=on
  gear : Outport  VectorParamsAs1DForOutWhenUnconnected=on
  wires:
  Constant3/1 -> "换档策略 "/2(PP)
  Constant6/1 -> "换档策略 "/5(DD)
  "换档策略 "/1(gear) -> gear/1
  Constant4/1 -> "换档策略 "/3(RR)
  Constant5/1 -> "换档策略 "/4(NN)
  v/1 -> "换档策略 "/1(v)

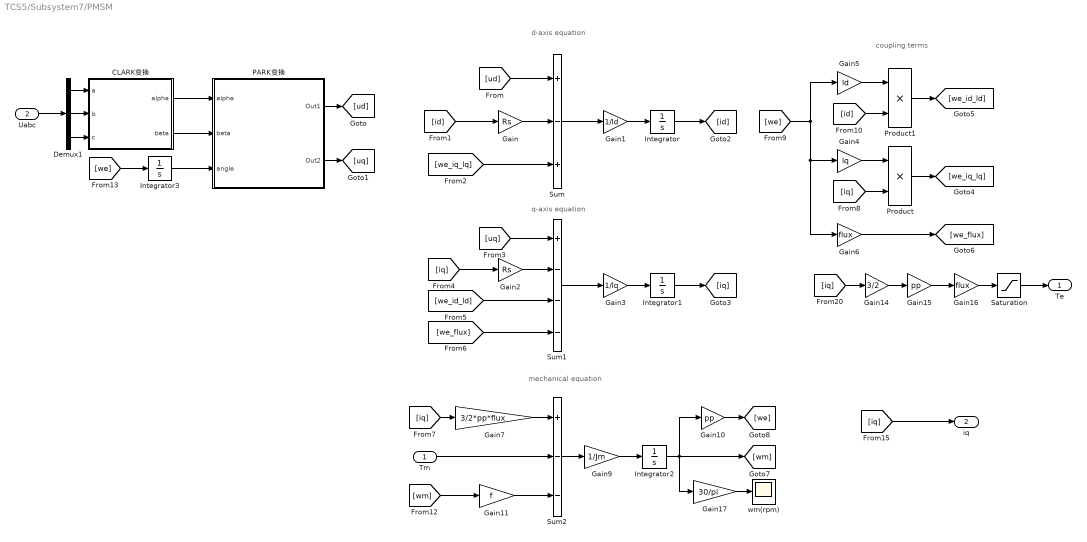
== system TCS5/Subsystem7/PMSM ==
  note: d-axis equation
  note: coupling terms
  note: q-axis equation
  note: mechanical equation
  Tm : Inport
  Uabc : Inport  Port=2
  CLARK变换 : Subsystem
  Demux1 : Demux  Outputs=3
  Gain : Gain  Gain=Rs
  Gain1 : Gain  Gain=1/ld
  Gain10 : Gain  Gain=pp
  Gain11 : Gain  Gain=f
  Gain14 : Gain  Gain=3/2
  Gain15 : Gain  Gain=pp
  Gain16 : Gain  Gain=flux
  Gain17 : Gain  Gain=30/pi
  Gain2 : Gain  Gain=Rs
  Gain3 : Gain  Gain=1/lq
  Gain4 : Gain  Gain=lq
  Gain5 : Gain  Gain=ld
  Gain6 : Gain  Gain=flux
  Gain7 : Gain  Gain=3/2*pp*flux
  Gain9 : Gain  Gain=1/Jm
  Integrator{,1..3} (4 alike) : Integrator
  PARK变换 : Subsystem
  Product : Product
  Product1 : Product
  Saturation : Saturate  UpperLimit=2000  LowerLimit=-2000
  Sum : Sum  Inputs=+-+
  Sum1 : Sum  Inputs=+---
  Sum2 : Sum  Inputs=+--
  wm(rpm) : Scope
  Te : Outport
  iq : Outport  Port=2
  wires:
  [iq] -> Product/2
  Integrator2/1 -> Gain17/1, [wm], Gain10/1
  [we_iq_lq] -> Sum/3
  [iq] -> Gain7/1
  Product1/1 -> [we_id_ld]
  Sum/1 -> Gain1/1
  Gain1/1 -> Integrator/1
  Gain2/1 -> Sum1/2
  Gain5/1 -> Product1/1
  Gain/1 -> Sum/2
  Gain3/1 -> Integrator1/1
  Sum1/1 -> Gain3/1
  [id] -> Product1/2
  Tm/1 -> Sum2/2
  [iq] -> Gain2/1
  Gain6/1 -> [we_flux]
  Gain9/1 -> Integrator2/1
  Product/1 -> [we_iq_lq]
  Gain7/1 -> Sum2/1
  Integrator1/1 -> [iq]
  Sum2/1 -> Gain9/1
  Gain4/1 -> Product/1
  [ud] -> Sum/1
  Gain10/1 -> [we]
  [we_flux] -> Sum1/4
  [we_id_ld] -> Sum1/3
  [we] -> Gain4/1, Gain6/1, Gain5/1
  [id] -> Gain/1
  [uq] -> Sum1/1
  Gain11/1 -> Sum2/3
  [wm] -> Gain11/1
  [iq] -> Gain14/1
  Gain14/1 -> Gain15/1
  Gain15/1 -> Gain16/1
  Gain17/1 -> wm(rpm)/1
  Integrator/1 -> [id]
  [iq] -> iq/1
  Gain16/1 -> Saturation/1
  Saturation/1 -> Te/1
  Demux1/1 -> CLARK变换/1(a)
  Uabc/1 -> Demux1/1
  Demux1/3 -> CLARK变换/3(c)
  Demux1/2 -> CLARK变换/2(b)
  CLARK变换/1(alpha) -> PARK变换/1(alpha)
  CLARK变换/2(beta) -> PARK变换/2(beta)
  [we] -> Integrator3/1
  Integrator3/1 -> PARK变换/3(angle)
  PARK变换/1(Out1) -> [ud]
  PARK变换/2(Out2) -> [uq]

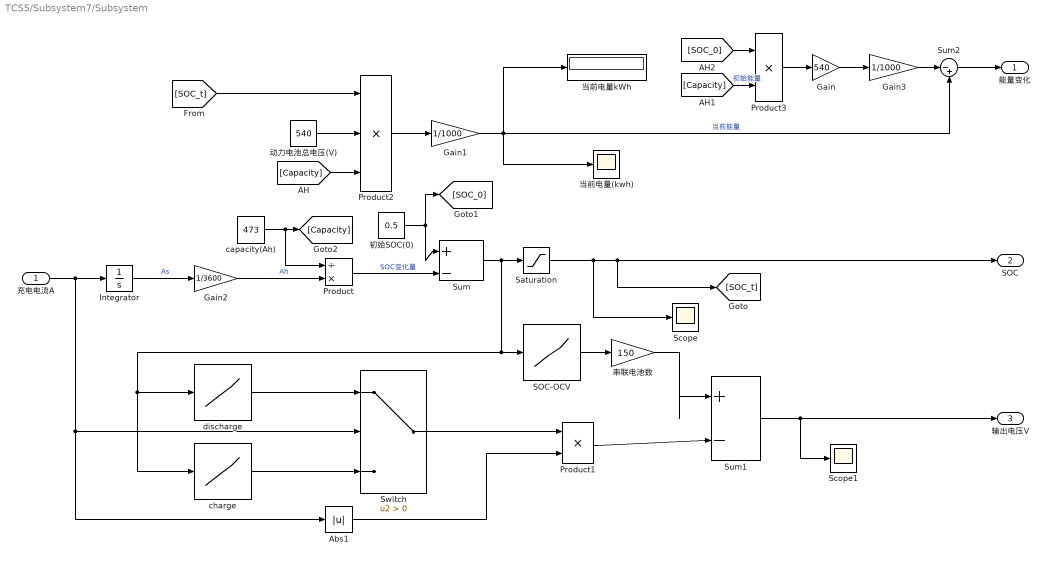
== system TCS5/Subsystem7/Subsystem ==
  充电电流A : Inport
  Abs1 : Abs
  Gain : Gain  Gain=540
  Gain1 : Gain  Gain=1/1000
  Gain2 : Gain  Gain=1/3600
  Gain3 : Gain  Gain=1/1000
  Integrator : Integrator
  Product : Product  Inputs=/*
  Product1 : Product
  Product2 : Product  Inputs=3
  Product3 : Product
  SOC-OCV : Lookup_n-D  NumberOfTableDimensions=1  BreakpointsForDimension1=[0,0.1,0.2,0.4,0.6,0.8,1]  Table=[3.31144,3.54994000000000013,3.63898,3.72908,3.8329600000000004,3.9771199999999998,4.131880000000001]  InternalRulePriority=Speed  RndMeth=Simplest  InputSameDT=on
  Saturation : Saturate  UpperLimit=1  LowerLimit=0
  Scope : Scope
  Scope1 : Scope
  Sum : Sum  Inputs=|+-
  Sum1 : Sum  Inputs=|+-
  Sum2 : Sum  Inputs=|-+
  Switch : Switch  Criteria=u2 > Threshold
  capacity(Ah) : Constant  Value=473
  charge : Lookup_n-D  NumberOfTableDimensions=1  BreakpointsForDimension1=[0,0.1,0.2,0.4,0.6,0.8,1]  Table=[0.02536,0.012695,0.0080907,0.006409000000000001,0.006565,0.0071812,0.0074386]  InternalRulePriority=Speed  RndMeth=Simplest  InputSameDT=on
  discharge : Lookup_n-D  NumberOfTableDimensions=1  BreakpointsForDimension1=[0,0.1,0.2,0.4,0.6,0.8,1]  Table=[0.02536,0.012695,0.0080907,0.006409000000000001,0.006565,0.0071812,0.0074386]  InternalRulePriority=Speed  RndMeth=Simplest  InputSameDT=on
  串联电池数 : Gain  Gain=150
  初始SOC(0) : Constant  Value=0.5
  动力电池总电压(V) : Constant  Value=540
  当前电量(kwh) : Scope
  当前电量kWh : Display
  能量变化 : Outport
  SOC : Outport  Port=2
  输出电压V : Outport  Port=3
  wires:
  Product2/1 -> Gain1/1
  初始SOC(0)/1 -> [SOC_0], Sum/1
  Saturation/1 -> Scope/1, SOC/1, [SOC_t]
  动力电池总电压(V)/1 -> Product2/2
  Product1/1 -> Sum1/2
  串联电池数/1 -> Sum1/1
  capacity(Ah)/1 -> [Capacity], Product/1
  Sum1/1 -> 输出电压V/1, Scope1/1
  charge/1 -> Switch/3
  Gain1/1 -> Sum2/2, 当前电量kWh/1, 当前电量(kwh)/1  "当前能量"
  SOC-OCV/1 -> 串联电池数/1
  充电电流A/1 -> Integrator/1, Abs1/1, Switch/2
  Sum/1 -> charge/1, discharge/1, SOC-OCV/1, Saturation/1
  Switch/1 -> Product1/1
  discharge/1 -> Switch/1
  [SOC_t] -> Product2/1
  Abs1/1 -> Product1/2
  [Capacity] -> Product2/3
  Product/1 -> Sum/2  "SOC变化量"
  Gain2/1 -> Product/2  "Ah"
  Integrator/1 -> Gain2/1  "As"
  Sum2/1 -> 能量变化/1
  Gain/1 -> Gain3/1
  Gain3/1 -> Sum2/1
  Product3/1 -> Gain/1
  [SOC_0] -> Product3/1
  [Capacity] -> Product3/2  "初始能量"

== system TCS5/Subsystem7/变速器模型 ==
  Tin : Inport  Unit=ft*lbf@torque
  Gear : Inport  Port=2  Unit=1
  Product : Product  SaturateOnIntegerOverflow=on  InputSameDT=on  OutDataTypeStr=Inherit: Same as first input
  Table : Lookup_n-D  NumberOfTableDimensions=1  BreakpointsForDimension1=[1 2 3 4]  Table=[7.93,3.53,1.74,1.00]  OutDataTypeStr=double  SaturateOnIntegerOverflow=on  InputSameDT=on  LockScale=on
  Tout : Outport  Unit=ft*lbf@torque
  wires:
  Table/1 -> Product/2
  Product/1 -> Tout/1
  Tin/1 -> Product/1
  Gear/1 -> Table/1

== system TCS5/Subsystem7/换挡逻辑 ==
  v : Inport
  Constant3 : Constant  Value=0
  Constant4 : Constant  Value=0
  Constant5 : Constant  Value=0
  Constant6 : Constant
  Rocker Switch : RockerSwitchBlock  WebBlockId=2700
      settings: Values={{'Off', 'On'}, [0 1]}
  Rocker Switch1 : RockerSwitchBlock  WebBlockId=2701
      settings: Values={{'Off', 'On'}, [0 1]}
  Rocker Switch2 : RockerSwitchBlock  WebBlockId=2702
      settings: Values={{'Off', 'On'}, [0 1]}
  Rocker Switch3 : RockerSwitchBlock  WebBlockId=2703
      settings: Values={{'Off', 'On'}, [0 1]}
  "换档策略 " : Stateflow chart  TreatAsAtomicUnit=on
  gear : Outport  VectorParamsAs1DForOutWhenUnconnected=on
  wires:
  Constant3/1 -> "换档策略 "/2(PP)
  Constant6/1 -> "换档策略 "/5(DD)
  "换档策略 "/1(gear) -> gear/1
  Constant4/1 -> "换档策略 "/3(RR)
  Constant5/1 -> "换档策略 "/4(NN)
  v/1 -> "换档策略 "/1(v)

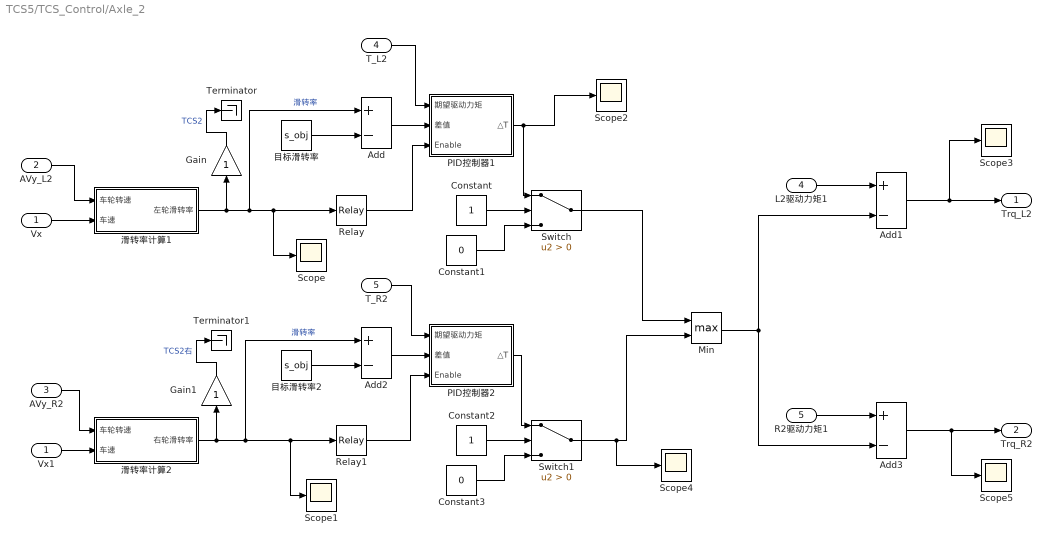
== system TCS5/TCS_Control/Axle_2 ==
  Vx : Inport
  AVy_L2 : Inport  Port=2
  AVy_R2 : Inport  Port=3
  T_L2 : Inport  Port=4
  T_R2 : Inport  Port=5
  Add{,1..3} (4 alike) : Sum  Inputs=+-
  Constant : Constant
  Constant1 : Constant  Value=0
  Constant2 : Constant
  Constant3 : Constant  Value=0
  Gain : Gain
  Gain1 : Gain
  L2驱动力矩1 : InportShadow  Port=4
  Min : MinMax  Function=max  Inputs=2
  PID控制器1 : Subsystem
  PID控制器2 : Subsystem
  R2驱动力矩1 : InportShadow  Port=5
  Relay : Relay  OnSwitchValue=0.13  OffSwitchValue=0.05
  Relay1 : Relay  OnSwitchValue=0.13  OffSwitchValue=0.05
  Scope{,1..5} (6 alike) : Scope
  Switch : Switch  Criteria=u2 > Threshold
  Switch1 : Switch  Criteria=u2 > Threshold
  Terminator : Terminator
  Terminator1 : Terminator
  Vx1 : InportShadow
  滑转率计算1 : Subsystem
  滑转率计算2 : Subsystem
  目标滑转率 : Constant  Value=s_obj
  目标滑转率2 : Constant  Value=s_obj
  Trq_L2 : Outport
  Trq_R2 : Outport  Port=2
  wires:
  PID控制器1/1(△T) -> Switch/1, Scope2/1
  Add3/1 -> Scope5/1, Trq_R2/1
  R2驱动力矩1/1 -> Add3/1
  目标滑转率/1 -> Add/2
  Constant1/1 -> Switch/3
  Min/1 -> Add3/2, Add1/2
  Add/1 -> PID控制器1/2(差值)
  目标滑转率2/1 -> Add2/2
  PID控制器2/1(△T) -> Switch1/1
  Add2/1 -> PID控制器2/2(差值)
  Switch1/1 -> Scope4/1, Min/2
  Relay1/1 -> PID控制器2/3(Enable)
  滑转率计算2/1(右轮滑转率) -> Gain1/1, Add2/1, Relay1/1, Scope1/1  "滑转率"
  Switch/1 -> Min/1
  Add1/1 -> Scope3/1, Trq_L2/1
  Constant3/1 -> Switch1/3
  Relay/1 -> PID控制器1/3(Enable)
  Vx/1 -> 滑转率计算1/2(车速)
  AVy_L2/1 -> 滑转率计算1/1(车轮转速)
  AVy_R2/1 -> 滑转率计算2/1(车轮转速)
  Vx1/1 -> 滑转率计算2/2(车速)
  T_R2/1 -> PID控制器2/1(期望驱动力矩)
  L2驱动力矩1/1 -> Add1/1
  T_L2/1 -> PID控制器1/1(期望驱动力矩)
  Gain/1 -> Terminator/1  "TCS2"
  滑转率计算1/1(左轮滑转率) -> Gain/1, Relay/1, Scope/1, Add/1  "滑转率"
  Gain1/1 -> Terminator1/1  "TCS2右"
  Constant/1 -> Switch/2
  Constant2/1 -> Switch1/2

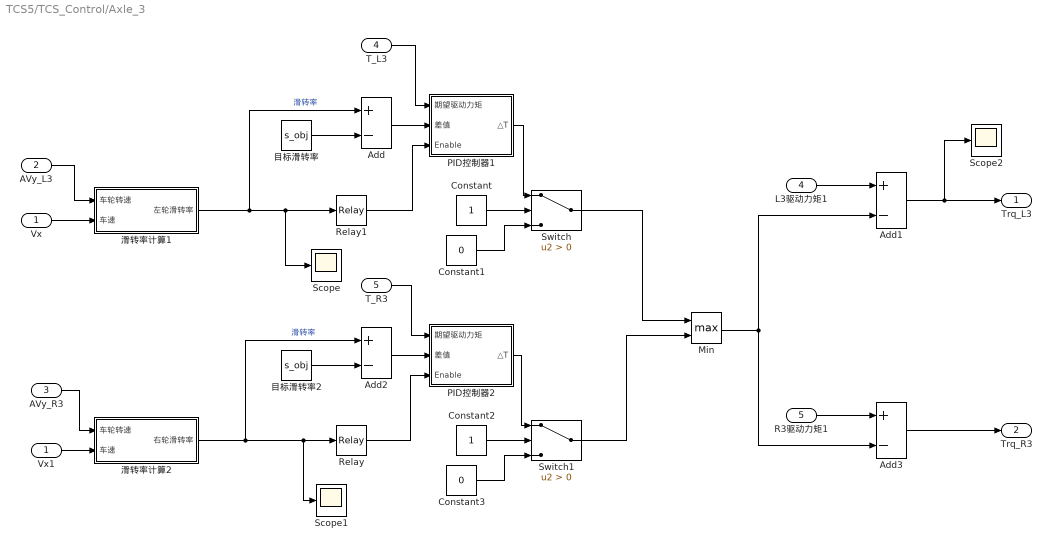
== system TCS5/TCS_Control/Axle_3 ==
  Vx : Inport
  AVy_L3 : Inport  Port=2
  AVy_R3 : Inport  Port=3
  T_L3 : Inport  Port=4
  T_R3 : Inport  Port=5
  Add{,1..3} (4 alike) : Sum  Inputs=+-
  Constant : Constant
  Constant1 : Constant  Value=0
  Constant2 : Constant
  Constant3 : Constant  Value=0
  L3驱动力矩1 : InportShadow  Port=4
  Min : MinMax  Function=max  Inputs=2
  PID控制器1 : Subsystem
  PID控制器2 : Subsystem
  R3驱动力矩1 : InportShadow  Port=5
  Relay : Relay  OnSwitchValue=0.13  OffSwitchValue=0.05
  Relay1 : Relay  OnSwitchValue=0.13  OffSwitchValue=0.05
  Scope : Scope
  Scope1 : Scope
  Scope2 : Scope
  Switch : Switch  Criteria=u2 > Threshold
  Switch1 : Switch  Criteria=u2 > Threshold
  Vx1 : InportShadow
  滑转率计算1 : Subsystem
  滑转率计算2 : Subsystem
  目标滑转率 : Constant  Value=s_obj
  目标滑转率2 : Constant  Value=s_obj
  Trq_L3 : Outport
  Trq_R3 : Outport  Port=2
  wires:
  PID控制器1/1(△T) -> Switch/1
  Add3/1 -> Trq_R3/1
  R3驱动力矩1/1 -> Add3/1
  目标滑转率/1 -> Add/2
  滑转率计算1/1(左轮滑转率) -> Scope/1, Relay1/1, Add/1  "滑转率"
  Constant1/1 -> Switch/3
  Min/1 -> Add3/2, Add1/2
  Add/1 -> PID控制器1/2(差值)
  目标滑转率2/1 -> Add2/2
  PID控制器2/1(△T) -> Switch1/1
  Add2/1 -> PID控制器2/2(差值)
  Switch1/1 -> Min/2
  Relay/1 -> PID控制器2/3(Enable)
  滑转率计算2/1(右轮滑转率) -> Scope1/1, Relay/1, Add2/1  "滑转率"
  Switch/1 -> Min/1
  Add1/1 -> Scope2/1, Trq_L3/1
  Constant3/1 -> Switch1/3
  Relay1/1 -> PID控制器1/3(Enable)
  Vx/1 -> 滑转率计算1/2(车速)
  AVy_L3/1 -> 滑转率计算1/1(车轮转速)
  AVy_R3/1 -> 滑转率计算2/1(车轮转速)
  Vx1/1 -> 滑转率计算2/2(车速)
  T_R3/1 -> PID控制器2/1(期望驱动力矩)
  L3驱动力矩1/1 -> Add1/1
  T_L3/1 -> PID控制器1/1(期望驱动力矩)
  Constant/1 -> Switch/2
  Constant2/1 -> Switch1/2

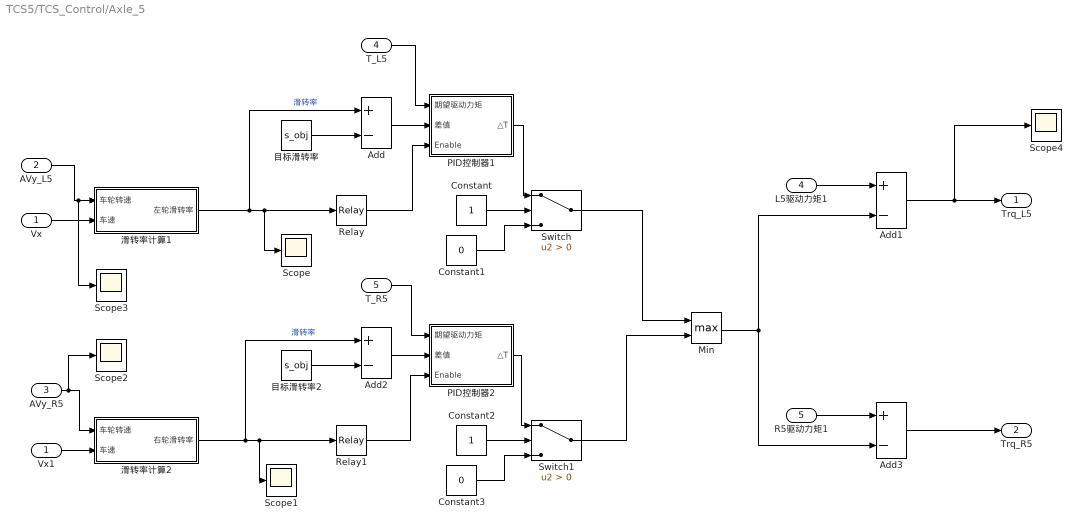
== system TCS5/TCS_Control/Axle_5 ==
  Vx : Inport
  AVy_L5 : Inport  Port=2
  AVy_R5 : Inport  Port=3
  T_L5 : Inport  Port=4
  T_R5 : Inport  Port=5
  Add{,1..3} (4 alike) : Sum  Inputs=+-
  Constant : Constant
  Constant1 : Constant  Value=0
  Constant2 : Constant
  Constant3 : Constant  Value=0
  L5驱动力矩1 : InportShadow  Port=4
  Min : MinMax  Function=max  Inputs=2
  PID控制器1 : Subsystem
  PID控制器2 : Subsystem
  R5驱动力矩1 : InportShadow  Port=5
  Relay : Relay  OnSwitchValue=0.13  OffSwitchValue=0.05
  Relay1 : Relay  OnSwitchValue=0.13  OffSwitchValue=0.05
  Scope{,1..4} (5 alike) : Scope
  Switch : Switch  Criteria=u2 > Threshold
  Switch1 : Switch  Criteria=u2 > Threshold
  Vx1 : InportShadow
  滑转率计算1 : Subsystem
  滑转率计算2 : Subsystem
  目标滑转率 : Constant  Value=s_obj
  目标滑转率2 : Constant  Value=s_obj
  Trq_L5 : Outport
  Trq_R5 : Outport  Port=2
  wires:
  PID控制器1/1(△T) -> Switch/1
  Add3/1 -> Trq_R5/1
  R5驱动力矩1/1 -> Add3/1
  目标滑转率/1 -> Add/2
  滑转率计算1/1(左轮滑转率) -> Scope/1, Relay/1, Add/1  "滑转率"
  Constant1/1 -> Switch/3
  Min/1 -> Add3/2, Add1/2
  Add/1 -> PID控制器1/2(差值)
  目标滑转率2/1 -> Add2/2
  PID控制器2/1(△T) -> Switch1/1
  Add2/1 -> PID控制器2/2(差值)
  Switch1/1 -> Min/2
  Relay1/1 -> PID控制器2/3(Enable)
  滑转率计算2/1(右轮滑转率) -> Scope1/1, Relay1/1, Add2/1  "滑转率"
  Switch/1 -> Min/1
  Add1/1 -> Scope4/1, Trq_L5/1
  Constant3/1 -> Switch1/3
  Relay/1 -> PID控制器1/3(Enable)
  Vx/1 -> 滑转率计算1/2(车速)
  AVy_R5/1 -> Scope2/1, 滑转率计算2/1(车轮转速)
  Vx1/1 -> 滑转率计算2/2(车速)
  T_R5/1 -> PID控制器2/1(期望驱动力矩)
  L5驱动力矩1/1 -> Add1/1
  T_L5/1 -> PID控制器1/1(期望驱动力矩)
  AVy_L5/1 -> Scope3/1, 滑转率计算1/1(车轮转速)
  Constant/1 -> Switch/2
  Constant2/1 -> Switch1/2

== system TCS5/TCS_Control/Estimate_Vx ==
  AVy_L4 : Inport
  AVy_R4 : Inport  Port=2
  Add : Sum
  Gain : Gain  Gain=pi/30
  Gain1 : Gain  Gain=3.6
  Gain2 : Gain  Gain=pi/30
  Gain3 : Gain  Gain=3.6
  Gain4 : Gain  Gain=0.5
  Product : Product
  Product1 : Product
  轮胎滚动半径 : Constant  Value=r
  轮胎滚动半径1 : Constant  Value=r
  Vx : Outport
  wires:
  Gain/1 -> Product/1
  Product1/1 -> Gain3/1
  Gain3/1 -> Add/2
  轮胎滚动半径/1 -> Product/2
  轮胎滚动半径1/1 -> Product1/2
  Add/1 -> Gain4/1
  Gain4/1 -> Vx/1
  Product/1 -> Gain1/1
  Gain1/1 -> Add/1
  Gain2/1 -> Product1/1
  AVy_R4/1 -> Gain2/1
  AVy_L4/1 -> Gain/1

== system TCS5/Subsystem5/PMSM/CLARK变换 ==
  a : Inport
  b : Inport  Port=2
  c : Inport  Port=3
  Fcn2 : Fcn  Expr=(2*u(1)-u(2)-u(3))/3
  Fcn3 : Fcn  Expr=sqrt(3)*(u(2)-u(3))/3
  Mux3 : Mux  Inputs=3
  alpha : Outport
  beta : Outport  Port=2
  wires:
  Mux3/1 -> Fcn3/1, Fcn2/1
  b/1 -> Mux3/2
  a/1 -> Mux3/1
  c/1 -> Mux3/3
  Fcn2/1 -> alpha/1
  Fcn3/1 -> beta/1

== system TCS5/Subsystem5/PMSM/PARK变换 ==
  alpha : Inport
  beta : Inport  Port=2
  angle : Inport  Port=3
  Fcn4 : Fcn  Expr=u(1)*cos(u(3))+u(2)*sin(u(3))
  Fcn5 : Fcn  Expr=-u(1)*sin(u(3))+u(2)*cos(u(3))
  Mux4 : Mux  Inputs=3
  Out1 : Outport
  Out2 : Outport  Port=2
  wires:
  Mux4/1 -> Fcn5/1, Fcn4/1
  beta/1 -> Mux4/2
  alpha/1 -> Mux4/1
  Fcn5/1 -> Out2/1
  angle/1 -> Mux4/3
  Fcn4/1 -> Out1/1

== system TCS5/Subsystem6/PMSM/CLARK变换 ==
  a : Inport
  b : Inport  Port=2
  c : Inport  Port=3
  Fcn2 : Fcn  Expr=(2*u(1)-u(2)-u(3))/3
  Fcn3 : Fcn  Expr=sqrt(3)*(u(2)-u(3))/3
  Mux3 : Mux  Inputs=3
  alpha : Outport
  beta : Outport  Port=2
  wires:
  Mux3/1 -> Fcn3/1, Fcn2/1
  b/1 -> Mux3/2
  a/1 -> Mux3/1
  c/1 -> Mux3/3
  Fcn2/1 -> alpha/1
  Fcn3/1 -> beta/1

== system TCS5/Subsystem6/PMSM/PARK变换 ==
  alpha : Inport
  beta : Inport  Port=2
  angle : Inport  Port=3
  Fcn4 : Fcn  Expr=u(1)*cos(u(3))+u(2)*sin(u(3))
  Fcn5 : Fcn  Expr=-u(1)*sin(u(3))+u(2)*cos(u(3))
  Mux4 : Mux  Inputs=3
  Out1 : Outport
  Out2 : Outport  Port=2
  wires:
  Mux4/1 -> Fcn5/1, Fcn4/1
  beta/1 -> Mux4/2
  alpha/1 -> Mux4/1
  Fcn5/1 -> Out2/1
  angle/1 -> Mux4/3
  Fcn4/1 -> Out1/1

== system TCS5/Subsystem7/PMSM/CLARK变换 ==
  a : Inport
  b : Inport  Port=2
  c : Inport  Port=3
  Fcn2 : Fcn  Expr=(2*u(1)-u(2)-u(3))/3
  Fcn3 : Fcn  Expr=sqrt(3)*(u(2)-u(3))/3
  Mux3 : Mux  Inputs=3
  alpha : Outport
  beta : Outport  Port=2
  wires:
  Mux3/1 -> Fcn3/1, Fcn2/1
  b/1 -> Mux3/2
  a/1 -> Mux3/1
  c/1 -> Mux3/3
  Fcn2/1 -> alpha/1
  Fcn3/1 -> beta/1

== system TCS5/Subsystem7/PMSM/PARK变换 ==
  alpha : Inport
  beta : Inport  Port=2
  angle : Inport  Port=3
  Fcn4 : Fcn  Expr=u(1)*cos(u(3))+u(2)*sin(u(3))
  Fcn5 : Fcn  Expr=-u(1)*sin(u(3))+u(2)*cos(u(3))
  Mux4 : Mux  Inputs=3
  Out1 : Outport
  Out2 : Outport  Port=2
  wires:
  Mux4/1 -> Fcn5/1, Fcn4/1
  beta/1 -> Mux4/2
  alpha/1 -> Mux4/1
  Fcn5/1 -> Out2/1
  angle/1 -> Mux4/3
  Fcn4/1 -> Out1/1

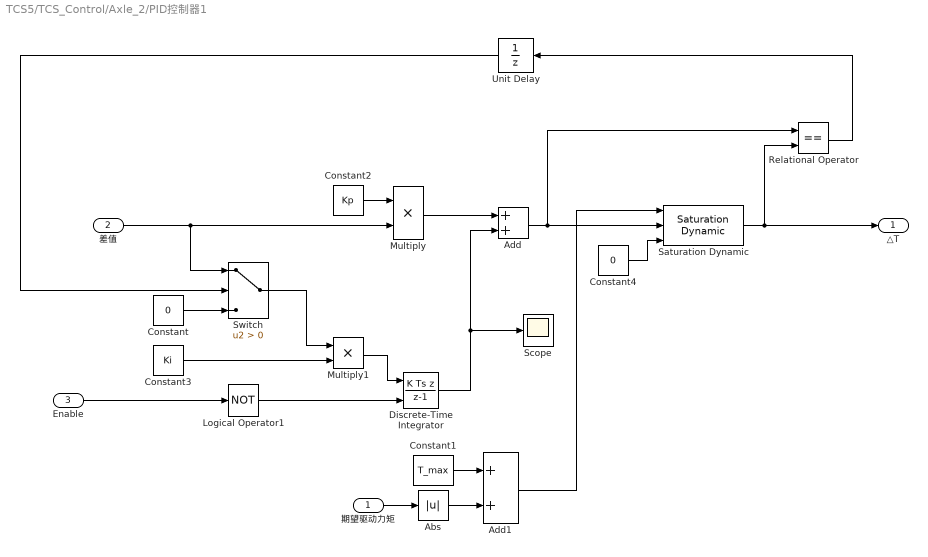
== system TCS5/TCS_Control/Axle_2/PID控制器1 ==
  期望驱动力矩 : Inport
  差值 : Inport  Port=2
  Enable : Inport  Port=3
  Abs : Abs
  Add : Sum
  Add1 : Sum
  Constant : Constant  Value=0  OutDataTypeStr=fixdt(1,16,5)
  Constant1 : Constant  Value=T_max
  Constant2 : Constant  Value=Kp
  Constant3 : Constant  Value=Ki
  Constant4 : Constant  Value=0
  Discrete-Time Integrator : DiscreteIntegrator  IntegratorMethod=Integration: Backward Euler  ExternalReset=level  SampleTime=-1  ICPrevOutput=DiscIntNeverNeededParam  ICPrevScaledInput=DiscIntNeverNeededParam
  Logical Operator1 : Logic  Operator=NOT  AllPortsSameDT=off  OutDataTypeStr=boolean
  Multiply : Product  OutDataTypeStr=fixdt(1,32,10)
  Multiply1 : Product  OutDataTypeStr=fixdt(1,32,10)
  Relational Operator : RelationalOperator  Operator===  OutDataTypeStr=boolean  RndMeth=Nearest
  Saturation Dynamic : simulink/Discontinuities/Saturation Dynamic  OutMin=[]  OutMax=[]  OutDataTypeStr=Inherit: Same as second input  OutDataType=fixdt(1, 16)  OutScaling=2^-10  DoSatur=off
  Scope : Scope
  Switch : Switch  Criteria=u2 > Threshold
  Unit Delay : UnitDelay  SampleTime=-1
  △T : Outport  VectorParamsAs1DForOutWhenUnconnected=on
  wires:
  Multiply/1 -> Add/1
  Discrete-Time Integrator/1 -> Scope/1, Add/2
  Enable/1 -> Logical Operator1/1
  Multiply1/1 -> Discrete-Time Integrator/1
  Constant3/1 -> Multiply1/2
  Relational Operator/1 -> Unit Delay/1
  Saturation Dynamic/1 -> Relational Operator/2, △T/1
  Constant2/1 -> Multiply/1
  Unit Delay/1 -> Switch/2
  差值/1 -> Switch/1, Multiply/2
  Add/1 -> Saturation Dynamic/2, Relational Operator/1
  Logical Operator1/1 -> Discrete-Time Integrator/2
  Switch/1 -> Multiply1/1
  Constant/1 -> Switch/3
  Constant1/1 -> Add1/1
  Add1/1 -> Saturation Dynamic/1
  期望驱动力矩/1 -> Abs/1
  Abs/1 -> Add1/2
  Constant4/1 -> Saturation Dynamic/3

== system TCS5/TCS_Control/Axle_2/PID控制器2 ==
  期望驱动力矩 : Inport
  差值 : Inport  Port=2
  Enable : Inport  Port=3
  Abs : Abs
  Add : Sum
  Add1 : Sum
  Constant : Constant  Value=0  OutDataTypeStr=fixdt(1,16,5)
  Constant1 : Constant  Value=T_max
  Constant2 : Constant  Value=Kp
  Constant3 : Constant  Value=Ki
  Constant4 : Constant  Value=0
  Discrete-Time Integrator : DiscreteIntegrator  IntegratorMethod=Integration: Backward Euler  ExternalReset=level  SampleTime=-1  ICPrevOutput=DiscIntNeverNeededParam  ICPrevScaledInput=DiscIntNeverNeededParam
  Logical Operator1 : Logic  Operator=NOT  AllPortsSameDT=off  OutDataTypeStr=boolean
  Multiply : Product  OutDataTypeStr=fixdt(1,32,10)
  Multiply1 : Product  OutDataTypeStr=fixdt(1,32,10)
  Relational Operator : RelationalOperator  Operator===  OutDataTypeStr=boolean  RndMeth=Nearest
  Saturation Dynamic : simulink/Discontinuities/Saturation Dynamic  OutMin=[]  OutMax=[]  OutDataTypeStr=Inherit: Same as second input  OutDataType=fixdt(1, 16)  OutScaling=2^-10  DoSatur=off
  Switch : Switch  Criteria=u2 > Threshold
  Unit Delay : UnitDelay  SampleTime=-1
  △T : Outport  VectorParamsAs1DForOutWhenUnconnected=on
  wires:
  Multiply/1 -> Add/1
  Discrete-Time Integrator/1 -> Add/2
  Enable/1 -> Logical Operator1/1
  Multiply1/1 -> Discrete-Time Integrator/1
  Constant3/1 -> Multiply1/2
  Relational Operator/1 -> Unit Delay/1
  Saturation Dynamic/1 -> Relational Operator/2, △T/1
  Constant2/1 -> Multiply/1
  Unit Delay/1 -> Switch/2
  差值/1 -> Switch/1, Multiply/2
  Add/1 -> Saturation Dynamic/2, Relational Operator/1
  Logical Operator1/1 -> Discrete-Time Integrator/2
  Switch/1 -> Multiply1/1
  Constant/1 -> Switch/3
  Constant1/1 -> Add1/1
  Add1/1 -> Saturation Dynamic/1
  期望驱动力矩/1 -> Abs/1
  Abs/1 -> Add1/2
  Constant4/1 -> Saturation Dynamic/3

== system TCS5/TCS_Control/Axle_2/滑转率计算1 ==
  车轮转速 : Inport
  车速 : Inport  Port=2
  Abs : Abs
  Add : Sum  Inputs=+-
  Add1 : Sum
  Constant : Constant  Value=0.001
  Divide : Product  Inputs=*/
  Gain : Gain  Gain=1/3.6
  Gain2 : Gain  Gain=pi/30
  Product : Product
  Saturation : Saturate  UpperLimit=1  LowerLimit=-1
  轮胎滚动半径 : Constant  Value=r
  左轮滑转率 : Outport  VectorParamsAs1DForOutWhenUnconnected=on
  wires:
  Saturation/1 -> 左轮滑转率/1
  Divide/1 -> Saturation/1
  轮胎滚动半径/1 -> Product/2
  Add/1 -> Divide/1
  Product/1 -> Abs/1, Add/1
  车速/1 -> Gain/1
  Gain/1 -> Add/2
  Gain2/1 -> Product/1
  车轮转速/1 -> Gain2/1
  Add1/1 -> Divide/2
  Constant/1 -> Add1/2
  Abs/1 -> Add1/1

== system TCS5/TCS_Control/Axle_2/滑转率计算2 ==
  车轮转速 : Inport
  车速 : Inport  Port=2
  Abs : Abs
  Add : Sum  Inputs=+-
  Add1 : Sum
  Constant : Constant  Value=0.001
  Divide : Product  Inputs=*/
  Gain : Gain  Gain=1/3.6
  Gain2 : Gain  Gain=pi/30
  Product : Product
  Saturation : Saturate  UpperLimit=1  LowerLimit=-1
  轮胎滚动半径 : Constant  Value=r
  右轮滑转率 : Outport  VectorParamsAs1DForOutWhenUnconnected=on
  wires:
  Saturation/1 -> 右轮滑转率/1
  Divide/1 -> Saturation/1
  轮胎滚动半径/1 -> Product/2
  Add/1 -> Divide/1
  Product/1 -> Abs/1, Add/1
  车速/1 -> Gain/1
  Gain/1 -> Add/2
  Gain2/1 -> Product/1
  车轮转速/1 -> Gain2/1
  Add1/1 -> Divide/2
  Constant/1 -> Add1/2
  Abs/1 -> Add1/1

== system TCS5/TCS_Control/Axle_3/PID控制器1 ==
  期望驱动力矩 : Inport
  差值 : Inport  Port=2
  Enable : Inport  Port=3
  Abs : Abs
  Add : Sum
  Add1 : Sum
  Constant : Constant  Value=0  OutDataTypeStr=fixdt(1,16,5)
  Constant1 : Constant  Value=T_max
  Constant2 : Constant  Value=Kp
  Constant3 : Constant  Value=Ki
  Constant4 : Constant  Value=0
  Discrete-Time Integrator : DiscreteIntegrator  IntegratorMethod=Integration: Backward Euler  ExternalReset=level  SampleTime=-1  ICPrevOutput=DiscIntNeverNeededParam  ICPrevScaledInput=DiscIntNeverNeededParam
  Logical Operator1 : Logic  Operator=NOT  AllPortsSameDT=off  OutDataTypeStr=boolean
  Multiply : Product  OutDataTypeStr=fixdt(1,32,10)
  Multiply1 : Product  OutDataTypeStr=fixdt(1,32,10)
  Relational Operator : RelationalOperator  Operator===  OutDataTypeStr=boolean  RndMeth=Nearest
  Saturation Dynamic : simulink/Discontinuities/Saturation Dynamic  OutMin=[]  OutMax=[]  OutDataTypeStr=Inherit: Same as second input  OutDataType=fixdt(1, 16)  OutScaling=2^-10  DoSatur=off
  Switch : Switch  Criteria=u2 > Threshold
  Unit Delay : UnitDelay  SampleTime=-1
  △T : Outport  VectorParamsAs1DForOutWhenUnconnected=on
  wires:
  Multiply/1 -> Add/1
  Discrete-Time Integrator/1 -> Add/2
  Enable/1 -> Logical Operator1/1
  Multiply1/1 -> Discrete-Time Integrator/1
  Constant3/1 -> Multiply1/2
  Relational Operator/1 -> Unit Delay/1
  Saturation Dynamic/1 -> Relational Operator/2, △T/1
  Constant2/1 -> Multiply/1
  Unit Delay/1 -> Switch/2
  差值/1 -> Switch/1, Multiply/2
  Add/1 -> Saturation Dynamic/2, Relational Operator/1
  Logical Operator1/1 -> Discrete-Time Integrator/2
  Switch/1 -> Multiply1/1
  Constant/1 -> Switch/3
  Constant1/1 -> Add1/1
  Add1/1 -> Saturation Dynamic/1
  期望驱动力矩/1 -> Abs/1
  Abs/1 -> Add1/2
  Constant4/1 -> Saturation Dynamic/3
